simulink model "EquavilentHalfBridge"  (R2018a)
settings: Solver=VariableStepAuto  StartTime=0.0  StopTime=1e-3  RelTol=1e-3
values from neighbouring files (symbols this model uses):
  Cds = Coss - Crss    [NumericCalcEx.m]    (also in mathematicalModel.m = 9e-12)
  Cgs = Ciss - Crss    [NumericCalcEx.m]    (also in mathematicalModel.m = 1e-12)
  Lload = 4e-6    (= 4e-06)    [StateSpaceHalfBridge.m]    (also in exStateSpaceHalf.m = 4e-05; mathematicalModel.m = 1e-06)
  Rgg = 3    [mathematicalModel.m]
  Rload = 100    [StateSpaceHalfBridge.m]    (also in exStateSpaceHalf.m = 10; mathematicalModel.m)
  Ron = 6    [mathematicalModel.m]
  Rrc = 10000    [mathematicalModel.m]
  Vth = 1.5    [mathematicalModel.m]
undefined symbols (not defined in the file or in its folder): U
libraries: cstblocks x2, simulink x2, dspmtrx3 x1
settings Model: Creator=enes_  LastModifiedBy=Furkan

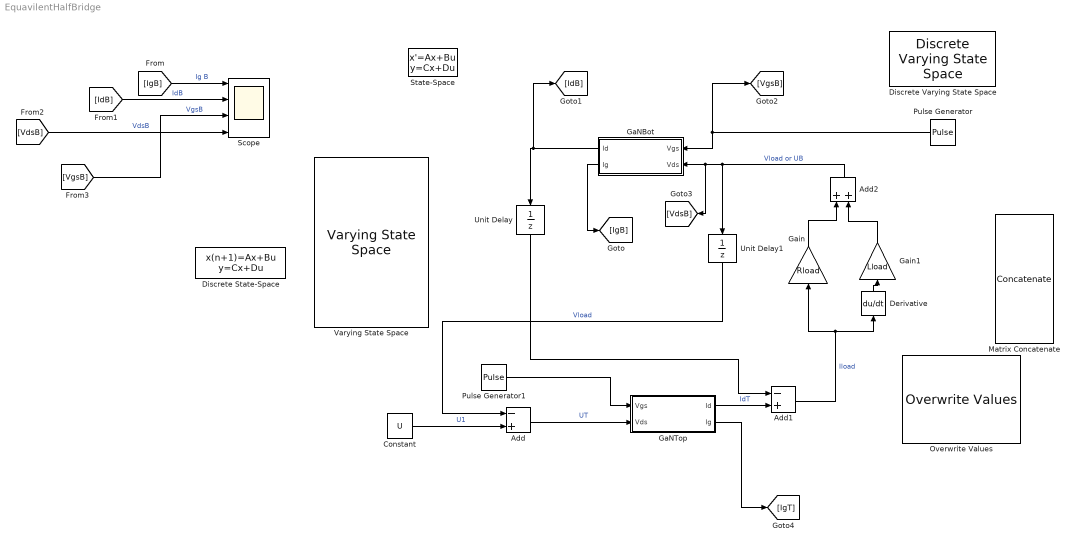
== system EquavilentHalfBridge ==
  Add : Sum  Inputs=-+
  Add1 : Sum  Inputs=-+
  Add2 : Sum
  Constant : Constant  Value=U
  Derivative : Derivative
  Discrete State-Space : DiscreteStateSpace  SampleTime=-1
  Discrete Varying State Space : cstblocks/Linear Parameter Varying/Discrete Varying State Space  x0=0  Ts=-1  OutputX=on  OutputDX=on
      settings: SourceProductName=Control System Toolbox  SourceProductBaseCode=CT
  GaNBot : Subsystem
  GaNTop : Subsystem
  Gain : Gain  Gain=Rload
  Gain1 : Gain  Gain=Lload
  Matrix Concatenate : Concatenate  NumInputs=4  Mode=Multidimensional array  ConcatenateDimension=2
  Overwrite Values : dspmtrx3/Overwrite Values  OverWriteDiag=Submatrix  valFrom2ndIP=Second input port  ConstValue=0  RowSpan=All rows  RowStartMode=First  RowStartIndex=1  RowEndMode=Last  RowEndIndex=1  ColSpan=All columns  ColStartMode=First  ColStartIndex=1  ColEndMode=Last  ColEndIndex=1  DiagSpan=Range of elements  DiagStartMode=Index  DiagStartIndex=2  DiagEndMode=Index  DiagEndIndex=4
      settings: SourceProductName=DSP System Toolbox  SourceProductBaseCode=DS
  Pulse Generator : DiscretePulseGenerator  PulseType=Time based  Period=1/10000  PulseWidth=50  PhaseDelay=1/20000
  Pulse Generator1 : DiscretePulseGenerator  PulseType=Time based  Period=1/10000  PulseWidth=50
  Scope : Scope  NumInputPorts=4
  State-Space : StateSpace  InitialCondition=0
  Unit Delay : UnitDelay  SampleTime=-1
  Unit Delay1 : UnitDelay  SampleTime=-1
  Varying State Space : cstblocks/Linear Parameter Varying/Varying State Space  x0=0  xNames=''  OutputX=on  OutputDX=on
      settings: SourceProductName=Control System Toolbox
  wires:
  Constant/1 -> Add/2  "U1"
  Add/1 -> GaNTop/2(Vds)  "UT"
  Pulse Generator1/1 -> GaNTop/1(Vgs)
  Unit Delay1/1 -> Add/1  "Vload"
  GaNTop/1(Id) -> Add1/2  "IdT"
  Add1/1 -> Derivative/1, Gain/1  "Iload"
  Derivative/1 -> Gain1/1
  Gain1/1 -> Add2/2
  Gain/1 -> Add2/1
  Add2/1 -> Unit Delay1/1, GaNBot/2(Vds), [VdsB]  "Vload or UB"
  Pulse Generator/1 -> GaNBot/1(Vgs), [VgsB]
  Unit Delay/1 -> Add1/1
  [IgB] -> Scope/1  "Ig B"
  [IdB] -> Scope/2  "IdB"
  [VdsB] -> Scope/4  "VdsB"
  [VgsB] -> Scope/3  "VgsB"
  GaNBot/2(Ig) -> [IgB]
  GaNBot/1(Id) -> [IdB], Unit Delay/1
  GaNTop/2(Ig) -> [IgT]

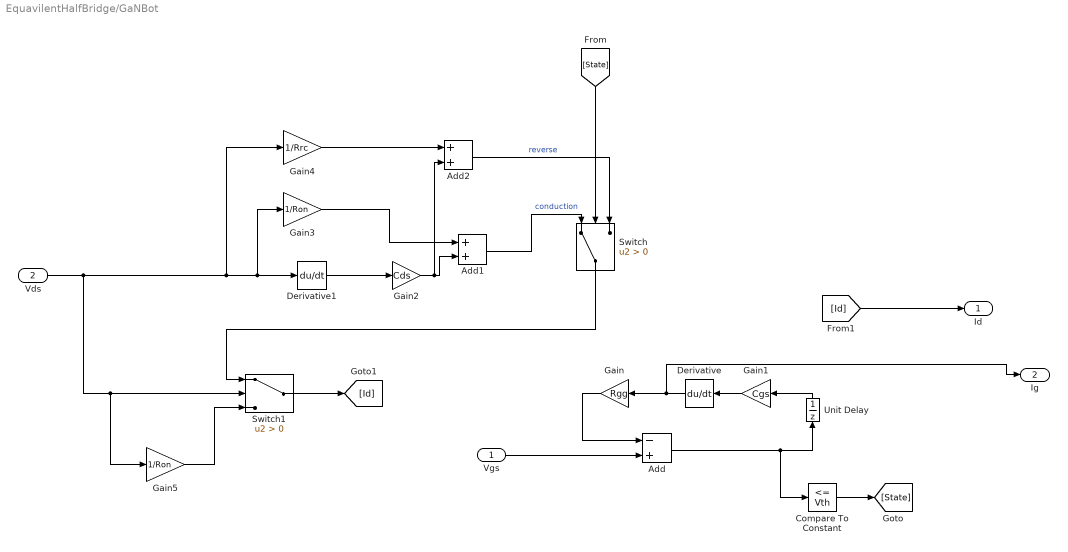
== system EquavilentHalfBridge/GaNBot ==
  Vgs : Inport
  Vds : Inport  Port=2
  Add : Sum  Inputs=-+
  Add1 : Sum
  Add2 : Sum
  Compare To Constant : simulink/Logic and Bit Operations/Compare To Constant  relop=<=  const=Vth  OutDataTypeStr=boolean
  Derivative : Derivative
  Derivative1 : Derivative
  Gain : Gain  Gain=Rgg
  Gain1 : Gain  Gain=Cgs
  Gain2 : Gain  Gain=Cds
  Gain3 : Gain  Gain=1/Ron
  Gain4 : Gain  Gain=1/Rrc
  Gain5 : Gain  Gain=1/Ron
  Switch : Switch  Criteria=u2 > Threshold
  Switch1 : Switch  Criteria=u2 > Threshold
  Unit Delay : UnitDelay  SampleTime=-1
  Id : Outport
  Ig : Outport  Port=2
  wires:
  Gain/1 -> Add/1
  Derivative1/1 -> Gain2/1
  Gain4/1 -> Add2/1
  [Id] -> Id/1
  Gain3/1 -> Add1/1
  Gain5/1 -> Switch1/3
  Add2/1 -> Switch/3  "reverse"
  Vds/1 -> Gain5/1, Switch1/2, Gain4/1, Gain3/1, Derivative1/1
  Add/1 -> Compare To Constant/1, Unit Delay/1
  Vgs/1 -> Add/2
  Compare To Constant/1 -> [State]
  Derivative/1 -> Ig/1, Gain/1
  Unit Delay/1 -> Gain1/1
  Add1/1 -> Switch/1  "conduction"
  [State] -> Switch/2
  Switch1/1 -> [Id]
  Gain2/1 -> Add2/2, Add1/2
  Gain1/1 -> Derivative/1
  Switch/1 -> Switch1/1

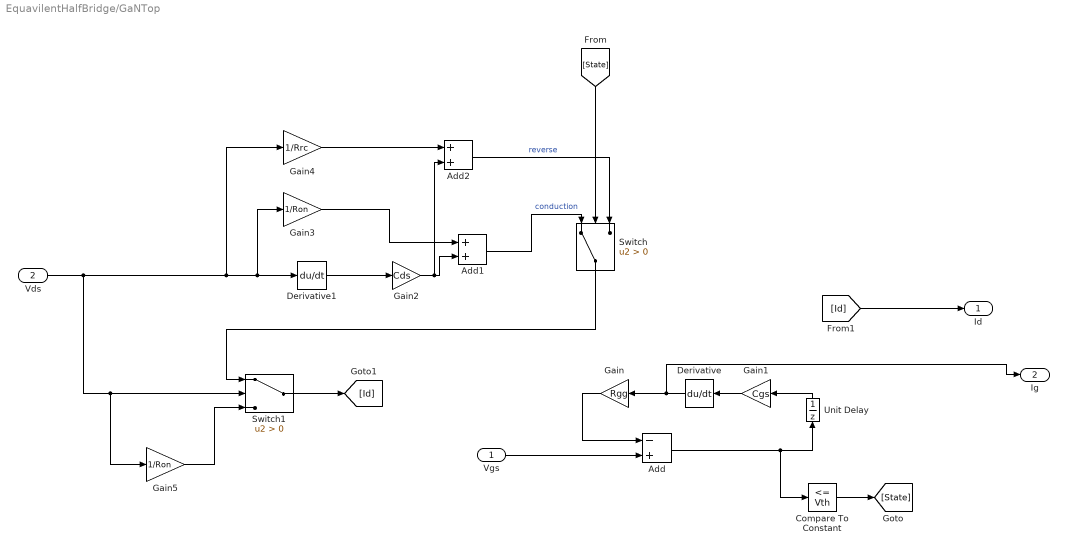
== system EquavilentHalfBridge/GaNTop ==
  Vgs : Inport
  Vds : Inport  Port=2
  Add : Sum  Inputs=-+
  Add1 : Sum
  Add2 : Sum
  Compare To Constant : simulink/Logic and Bit Operations/Compare To Constant  relop=<=  const=Vth  OutDataTypeStr=boolean
  Derivative : Derivative
  Derivative1 : Derivative
  Gain : Gain  Gain=Rgg
  Gain1 : Gain  Gain=Cgs
  Gain2 : Gain  Gain=Cds
  Gain3 : Gain  Gain=1/Ron
  Gain4 : Gain  Gain=1/Rrc
  Gain5 : Gain  Gain=1/Ron
  Switch : Switch  Criteria=u2 > Threshold
  Switch1 : Switch  Criteria=u2 > Threshold
  Unit Delay : UnitDelay  SampleTime=-1
  Id : Outport
  Ig : Outport  Port=2
  wires:
  Vgs/1 -> Add/2
  Gain1/1 -> Derivative/1
  Add/1 -> Compare To Constant/1, Unit Delay/1
  Derivative/1 -> Ig/1, Gain/1
  Unit Delay/1 -> Gain1/1
  Compare To Constant/1 -> [State]
  [State] -> Switch/2
  Gain/1 -> Add/1
  Vds/1 -> Gain5/1, Switch1/2, Gain4/1, Gain3/1, Derivative1/1
  Derivative1/1 -> Gain2/1
  Gain2/1 -> Add2/2, Add1/2
  Gain3/1 -> Add1/1
  Add1/1 -> Switch/1  "conduction"
  Gain4/1 -> Add2/1
  Add2/1 -> Switch/3  "reverse"
  Switch/1 -> Switch1/1
  Gain5/1 -> Switch1/3
  Switch1/1 -> [Id]
  [Id] -> Id/1
